simulink model "test_descramble_x_eng_reord"  (Simulink 6.2)
settings: Solver=ode45  StartTime=0.0  StopTime=10000  RelTol=1e-3
undefined symbols (not defined in the file or in its folder): BitWidth, cmult_4bit_em
libraries: xbsIndex_r3 x370, casper_library x29, xps_library x9, simulink x1
(part 2 of 3)

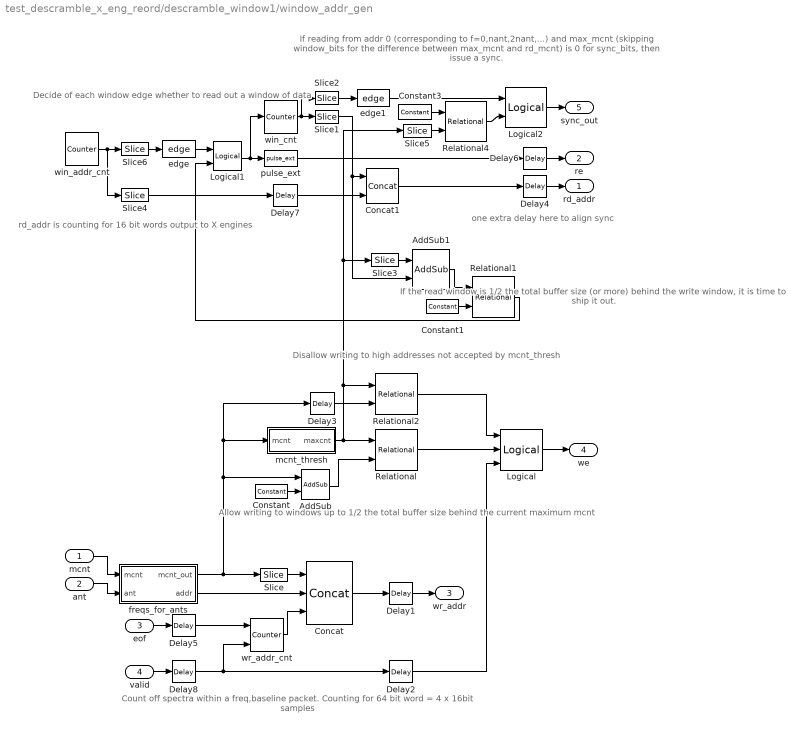
== system test_descramble_x_eng_reord/descramble_window1/window_addr_gen ==
  note: one extra delay
      | here to align sync
  note: If reading from addr 0 (corresponding to f=0,nant,2nant,...)
      | and max_mcnt (skipping window_bits for the difference
      | between max_mcnt and rd_mcnt) is 0 for sync_bits, then
      | issue a sync.
  note: Allow writing to windows
      | up to 1/2 the total buffer size
      |  behind the current maximum mcnt
  note: Count off spectra
      | within a freq,baseline
      | packet.  Counting for
      | 64 bit word = 4 x 16bit samples
  note: Decide of each window
      | edge whether to read
      | out a window of data
  note: If the read window is 1/2
      | the total buffer size (or more)
      | behind the write window,
      | it is time to ship it out.
  note: rd_addr is counting for
      | 16 bit words output to
      | X engines
  note: Disallow writing to high addresses
      | not accepted by mcnt_thresh
  mcnt : Inport  Port=1  LatchInput=off
  ant : Inport  Port=2  LatchInput=off
  eof : Inport  Port=3  LatchInput=off
  valid : Inport  Port=4  LatchInput=off
  AddSub : xbsIndex_r3/AddSub  mode=Addition  precision=User Defined  arith_type=Unsigned  n_bits=48 - ant_bits  bin_pt=0  quantization=Truncate  overflow=Wrap  latency=2  explicit_period=off  period=1  use_carryin=off  use_carryout=off  en=off  dbl_ovrd=off  show_param=off  use_core=on  pipeline=off  use_rpm=on  gen_core=off
      settings: xl_area=[0, 0, 0, 0, 0, 0, 0]
  AddSub1 : xbsIndex_r3/AddSub  mode=Subtraction  precision=User Defined  arith_type=Unsigned  n_bits=window_bits  bin_pt=0  quantization=Truncate  overflow=Wrap  latency=2  explicit_period=off  period=1  use_carryin=off  use_carryout=off  en=off  dbl_ovrd=off  show_param=off  use_core=on  pipeline=off  use_rpm=on  gen_core=off
      settings: xl_area=[0, 0, 0, 0, 0, 0, 0]
  Concat : xbsIndex_r3/Concat  num_inputs=3  explicit_period=off  period=1  dbl_ovrd=off
  Concat1 : xbsIndex_r3/Concat  num_inputs=2  explicit_period=off  period=1  dbl_ovrd=off
  Constant : xbsIndex_r3/Constant  const=2^(window_bits - 1)  equ=P=C  arith_type=Unsigned  n_bits=48 - ant_bits  bin_pt=0  opselect=C  inp2=PCIN>>17  opr=+  inp1=P  carry=CIN  iostate=0  explicit_period=on  period=1  dbl_ovrd=off
  Constant1 : xbsIndex_r3/Constant  const=2^(window_bits - 1)  equ=P=C  arith_type=Unsigned  n_bits=window_bits  bin_pt=0  opselect=C  inp2=PCIN>>17  opr=+  inp1=P  carry=CIN  iostate=0  explicit_period=on  period=1  dbl_ovrd=off
  Constant3 : xbsIndex_r3/Constant  const=0  equ=P=C  arith_type=Unsigned  n_bits=sync_bits - x_int_bits - ant_bits - window_bits  bin_pt=0  opselect=C  inp2=PCIN>>17  opr=+  inp1=P  carry=CIN  iostate=0  explicit_period=on  period=1  dbl_ovrd=off
  Delay1 : xbsIndex_r3/Delay  latency=3  reg_retiming=off  explicit_period=off  period=1  en=off  accept_only_valid=off  init_zero=on  dbl_ovrd=off  show_param=off
      settings: xl_area=[0, 0, 0, 0, 0, 0, 0]
  Delay2 : xbsIndex_r3/Delay  latency=3  reg_retiming=off  explicit_period=off  period=1  en=off  accept_only_valid=off  init_zero=on  dbl_ovrd=off  show_param=off
      settings: xl_area=[0, 0, 0, 0, 0, 0, 0]
  Delay3 : xbsIndex_r3/Delay  latency=2  reg_retiming=off  explicit_period=off  period=1  en=off  accept_only_valid=off  init_zero=on  dbl_ovrd=off  show_param=off
      settings: xl_area=[0, 0, 0, 0, 0, 0, 0]
  Delay{4..8} (5 alike) : xbsIndex_r3/Delay  latency=1  reg_retiming=off  explicit_period=off  period=1  en=off  accept_only_valid=off  init_zero=on  dbl_ovrd=off  show_param=off
      settings: xl_area=[0, 0, 0, 0, 0, 0, 0]
  Logical : xbsIndex_r3/Logical  logical_function=AND  inputs=3  precision=Full  arith_type=Unsigned  n_bits=8  bin_pt=2  align_bp=on  latency=0  explicit_period=off  period=1  en=off  dbl_ovrd=off  show_param=off
      settings: xl_area=[0, 0, 0, 0, 0, 0, 0]
  Logical1 : xbsIndex_r3/Logical  logical_function=AND  inputs=2  precision=Full  arith_type=Unsigned  n_bits=8  bin_pt=2  align_bp=on  latency=0  explicit_period=off  period=1  en=off  dbl_ovrd=off  show_param=off
      settings: xl_area=[0, 0, 0, 0, 0, 0, 0]
  Logical2 : xbsIndex_r3/Logical  logical_function=AND  inputs=2  precision=Full  arith_type=Unsigned  n_bits=8  bin_pt=2  align_bp=on  latency=0  explicit_period=off  period=1  en=off  dbl_ovrd=off  show_param=off
      settings: xl_area=[0, 0, 0, 0, 0, 0, 0]
  Relational : xbsIndex_r3/Relational  mode=a<b  latency=1  explicit_period=off  period=1  en=off  dbl_ovrd=off  show_param=off
      settings: xl_area=[0, 0, 0, 0, 0, 0, 0]
  Relational1 : xbsIndex_r3/Relational  mode=a>=b  latency=1  explicit_period=on  period=1  en=off  dbl_ovrd=off  show_param=off
      settings: xl_area=[0, 0, 0, 0, 0, 0, 0]
  Relational2 : xbsIndex_r3/Relational  mode=a>=b  latency=1  explicit_period=off  period=1  en=off  dbl_ovrd=off  show_param=off
      settings: xl_area=[0, 0, 0, 0, 0, 0, 0]
  Relational4 : xbsIndex_r3/Relational  mode=a=b  latency=1  explicit_period=off  period=1  en=off  dbl_ovrd=off  show_param=off
      settings: xl_area=[0, 0, 0, 0, 0, 0, 0]
  Slice : xbsIndex_r3/Slice  mode=Lower Bit Location + Width  nbits=window_bits  bit1=0  base1=MSB of Input  bit0=0  base0=LSB of Input  boolean_output=off  explicit_period=off  period=1  dbl_ovrd=off
  Slice1 : xbsIndex_r3/Slice  mode=Lower Bit Location + Width  nbits=window_bits  bit1=0  base1=MSB of Input  bit0=0  base0=LSB of Input  boolean_output=off  explicit_period=off  period=1  dbl_ovrd=off
  Slice2 : xbsIndex_r3/Slice  mode=Upper Bit Location + Width  nbits=1  bit1=0  base1=MSB of Input  bit0=0  base0=LSB of Input  boolean_output=on  explicit_period=off  period=1  dbl_ovrd=off
  Slice3 : xbsIndex_r3/Slice  mode=Lower Bit Location + Width  nbits=window_bits  bit1=0  base1=MSB of Input  bit0=0  base0=LSB of Input  boolean_output=off  explicit_period=off  period=1  dbl_ovrd=off
  Slice4 : xbsIndex_r3/Slice  mode=Lower Bit Location + Width  nbits=x_int_bits + ant_bits  bit1=0  base1=MSB of Input  bit0=0  base0=LSB of Input  boolean_output=off  explicit_period=off  period=1  dbl_ovrd=off
  Slice5 : xbsIndex_r3/Slice  mode=Two Bit Locations  nbits=window_bits  bit1=sync_bits - x_int_bits - ant_bits - 1  base1=LSB of Input  bit0=window_bits  base0=LSB of Input  boolean_output=off  explicit_period=off  period=1  dbl_ovrd=off
  Slice6 : xbsIndex_r3/Slice  mode=Upper Bit Location + Width  nbits=1  bit1=0  base1=MSB of Input  bit0=0  base0=LSB of Input  boolean_output=on  explicit_period=off  period=1  dbl_ovrd=off
  edge : casper_library/Misc/edge
  edge1 : casper_library/Misc/edge
  freqs_for_ants : Subsystem
  mcnt_thresh : Subsystem
  pulse_ext : casper_library/Misc/pulse_ext  pulse_len=2^(x_int_bits + ant_bits)
  win_addr_cnt : xbsIndex_r3/Counter  cnt_type=Free Running  n_bits=x_int_bits + ant_bits + 1  bin_pt=0  arith_type=Unsigned  start_count=0  cnt_to=Inf  cnt_by_val=1  operation=Up  explicit_period=off  period=1  load_pin=off  rst=off  en=off  dbl_ovrd=off  show_param=off  use_rpm=on  gen_core=off
      settings: xl_area=[0, 0, 0, 0, 0, 0, 0]
  win_cnt : xbsIndex_r3/Counter  cnt_type=Free Running  n_bits=window_bits + 1  bin_pt=0  arith_type=Unsigned  start_count=0  cnt_to=Inf  cnt_by_val=1  operation=Up  explicit_period=off  period=1  load_pin=off  rst=off  en=on  dbl_ovrd=off  show_param=off  use_rpm=on  gen_core=off
      settings: xl_area=[0, 0, 0, 0, 0, 0, 0]
  wr_addr_cnt : xbsIndex_r3/Counter  cnt_type=Free Running  n_bits=x_int_bits - 2  bin_pt=0  arith_type=Unsigned  start_count=0  cnt_to=Inf  cnt_by_val=1  operation=Up  explicit_period=off  period=1  load_pin=off  rst=on  en=on  dbl_ovrd=off  show_param=off  use_rpm=on  gen_core=off
      settings: xl_area=[0, 0, 0, 0, 0, 0, 0]
  rd_addr : Outport
  re : Outport  Port=2
  wr_addr : Outport  Port=3
  we : Outport  Port=4
  sync_out : Outport  Port=5
  wires:
  pulse_ext/1 -> Delay6/1
  Concat1/1 -> Delay4/1
  Delay7/1 -> Concat1/2
  Slice2/1 -> edge1/1
  Slice1/1 -> Concat1/1, AddSub1/2
  Slice4/1 -> Delay7/1
  freqs_for_ants/1(mcnt_out) -> Delay3/1, mcnt_thresh/1(mcnt), AddSub/1, Slice/1
  edge/1 -> Logical1/1
  Slice6/1 -> edge/1
  win_addr_cnt/1 -> Slice4/1, Slice6/1
  Delay6/1 -> re/1
  Delay4/1 -> rd_addr/1
  Relational1/1 -> Logical1/2
  Logical2/1 -> sync_out/1
  Relational4/1 -> Logical2/2
  Slice5/1 -> Relational4/2
  Constant3/1 -> Relational4/1
  edge1/1 -> Logical2/1
  Delay3/1 -> Relational2/2
  Relational2/1 -> Logical/1
  mcnt_thresh/1(maxcnt) -> Relational2/1, Slice5/1, Slice3/1, Relational/1
  Constant/1 -> AddSub/2
  mcnt/1 -> freqs_for_ants/1(mcnt)
  AddSub/1 -> Relational/2
  Slice/1 -> Concat/1
  freqs_for_ants/2(addr) -> Concat/2
  Concat/1 -> Delay1/1
  Delay1/1 -> wr_addr/1
  ant/1 -> freqs_for_ants/2(ant)
  wr_addr_cnt/1 -> Concat/3
  valid/1 -> Delay8/1
  eof/1 -> Delay5/1
  Relational/1 -> Logical/2
  Logical/1 -> we/1
  Delay2/1 -> Logical/3
  Logical1/1 -> win_cnt/1, pulse_ext/1
  Slice3/1 -> AddSub1/1
  win_cnt/1 -> Slice2/1, Slice1/1
  AddSub1/1 -> Relational1/1
  Constant1/1 -> Relational1/2
  Delay5/1 -> wr_addr_cnt/1
  Delay8/1 -> wr_addr_cnt/2, Delay2/1

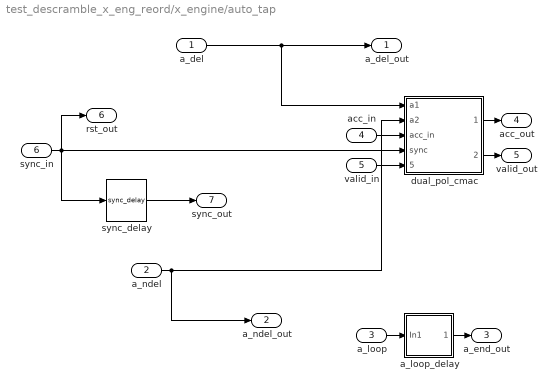
== system test_descramble_x_eng_reord/x_engine/auto_tap ==
  a_del : Inport  Port=1  LatchInput=off
  a_ndel : Inport  Port=2  LatchInput=off
  a_loop : Inport  Port=3  LatchInput=off
  acc_in : Inport  Port=4  LatchInput=off
  valid_in : Inport  Port=5  LatchInput=off
  sync_in : Inport  Port=6  LatchInput=off
  a_loop_delay : Subsystem  BlockChoice=delay_bram
      link override delay_bram: DelayLen=(acc_len - 1)*ceil(n_ants/2) + ceil(n_ants/2)-floor(n_ants/2)  bram_latency=bram_latency
      link override delay_bram/Constant2: equ=P=C
      settings: AttributesFormatString=%<BlockChoice>  TemplateBlock=casper_library/Delays/delay  MemberBlocks=delay_bram,delay_slr
  dual_pol_cmac : Subsystem
  sync_delay : casper_library/Delays/sync_delay  DelayLen=add_latency + mult_latency + acc_len + floor(n_ants/2 + 1) + 1
      link override Constant: equ=P=C
      link override Constant1: equ=P=C
      link override Constant2: equ=P=C
      link override Constant3: equ=P=C
  a_del_out : Outport
  a_ndel_out : Outport  Port=2
  a_end_out : Outport  Port=3
  acc_out : Outport  Port=4
  valid_out : Outport  Port=5
  rst_out : Outport  Port=6
  sync_out : Outport  Port=7
  wires:
  sync_in/1 -> sync_delay/1, dual_pol_cmac/4(sync), rst_out/1
  a_del/1 -> dual_pol_cmac/1(a1), a_del_out/1
  dual_pol_cmac/1(acc_out) -> acc_out/1
  acc_in/1 -> dual_pol_cmac/3(acc_in)
  dual_pol_cmac/2(valid_out) -> valid_out/1
  valid_in/1 -> dual_pol_cmac/5(valid_in)
  a_ndel/1 -> dual_pol_cmac/2(a2), a_ndel_out/1
  a_loop/1 -> a_loop_delay/1(In1)
  a_loop_delay/1(Out1) -> a_end_out/1
  sync_delay/1 -> sync_out/1

== system test_descramble_x_eng_reord/descramble_window1/window_addr_gen/freqs_for_ants ==
  note: skip bits of mcnt
      | for frequencies sent
      | to other X engines
  note: If correlator is configured to do fewer antennas, then more
      | frequencies come.  We just pretend here that the extra
      | frequencies are other antennas.
  mcnt : Inport  Port=1  LatchInput=off
  ant : Inport  Port=2  LatchInput=off
  Concat3 : xbsIndex_r3/Concat  num_inputs=2  explicit_period=off  period=1  dbl_ovrd=off
  Slice1 : xbsIndex_r3/Slice  mode=Lower Bit Location + Width  nbits=ant_bits  bit1=0  base1=MSB of Input  bit0=0  base0=LSB of Input  boolean_output=off  explicit_period=off  period=1  dbl_ovrd=off
  Slice14 : xbsIndex_r3/Slice  mode=Two Bit Locations  nbits=ant_bits  bit1=0  base1=MSB of Input  bit0=ant_bits  base0=LSB of Input  boolean_output=off  explicit_period=off  period=1  dbl_ovrd=off
  Slice18 : xbsIndex_r3/Slice  mode=Lower Bit Location + Width  nbits=ant_bits  bit1=0  base1=MSB of Input  bit0=0  base0=LSB of Input  boolean_output=off  explicit_period=off  period=1  dbl_ovrd=off
  Slice19 : xbsIndex_r3/Slice  mode=Two Bit Locations  nbits=48  bit1=0  base1=MSB of Input  bit0=ant_bits  base0=LSB of Input  boolean_output=off  explicit_period=off  period=1  dbl_ovrd=off
  mcnt_out : Outport
  addr : Outport  Port=2
  wires:
  Slice19/1 -> mcnt_out/1
  Slice18/1 -> addr/1
  Slice14/1 -> Concat3/1
  Slice1/1 -> Concat3/2
  Concat3/1 -> Slice19/1, Slice18/1
  ant/1 -> Slice1/1
  mcnt/1 -> Slice14/1

== system test_descramble_x_eng_reord/descramble_window1/window_addr_gen/mcnt_thresh ==
  note: timeout of a bad
      | master count
      | in ~2^20 clocks
  note: capture any new mcnts
      | which are within 1/4 buffer
      | of the previous mcnt.
      | This prevents locking onto
      | bad mcnts
  mcnt : Inport  Port=1  LatchInput=off
  AddSub : xbsIndex_r3/AddSub  mode=Addition  precision=User Defined  arith_type=Unsigned  n_bits=48 - ant_bits  bin_pt=0  quantization=Truncate  overflow=Wrap  latency=2  explicit_period=off  period=1  use_carryin=off  use_carryout=off  en=off  dbl_ovrd=off  show_param=off  use_core=on  pipeline=off  use_rpm=on  gen_core=off
      settings: xl_area=[0, 0, 0, 0, 0, 0, 0]
  Constant : xbsIndex_r3/Constant  const=2^(window_bits - 2)  equ=P=C  arith_type=Unsigned  n_bits=48 - ant_bits  bin_pt=0  opselect=C  inp2=PCIN>>17  opr=+  inp1=P  carry=CIN  iostate=0  explicit_period=on  period=1  dbl_ovrd=off
  Counter : xbsIndex_r3/Counter  cnt_type=Free Running  n_bits=21  bin_pt=0  arith_type=Unsigned  start_count=0  cnt_to=Inf  cnt_by_val=1  operation=Up  explicit_period=on  period=1  load_pin=off  rst=on  en=off  dbl_ovrd=off  show_param=off  use_rpm=on  gen_core=off
      settings: xl_area=[0, 0, 0, 0, 0, 0, 0]
  Delay : xbsIndex_r3/Delay  latency=2  reg_retiming=off  explicit_period=off  period=1  en=off  accept_only_valid=off  init_zero=on  dbl_ovrd=off  show_param=off
      settings: xl_area=[0, 0, 0, 0, 0, 0, 0]
  Delay1 : xbsIndex_r3/Delay  latency=1  reg_retiming=off  explicit_period=off  period=1  en=off  accept_only_valid=off  init_zero=on  dbl_ovrd=off  show_param=off
      settings: xl_area=[0, 0, 0, 0, 0, 0, 0]
  Logical : xbsIndex_r3/Logical  logical_function=AND  inputs=2  precision=Full  arith_type=Unsigned  n_bits=8  bin_pt=2  align_bp=on  latency=0  explicit_period=off  period=1  en=off  dbl_ovrd=off  show_param=off
      settings: xl_area=[0, 0, 0, 0, 0, 0, 0]
  Logical1 : xbsIndex_r3/Logical  logical_function=OR  inputs=2  precision=Full  arith_type=Unsigned  n_bits=8  bin_pt=2  align_bp=on  latency=0  explicit_period=off  period=1  en=off  dbl_ovrd=off  show_param=off
      settings: xl_area=[0, 0, 0, 0, 0, 0, 0]
  Register : xbsIndex_r3/Register  init=0  reg_only_valid=off  explicit_period=on  period=1  rst=off  en=on  out_en=off  dbl_ovrd=off  show_param=off
      settings: xl_area=[0, 0, 0, 0, 0, 0, 0]
  Relational : xbsIndex_r3/Relational  mode=a>b  latency=1  explicit_period=off  period=1  en=off  dbl_ovrd=off  show_param=off
      settings: xl_area=[0, 0, 0, 0, 0, 0, 0]
  Relational1 : xbsIndex_r3/Relational  mode=a<b  latency=1  explicit_period=off  period=1  en=off  dbl_ovrd=off  show_param=off
      settings: xl_area=[0, 0, 0, 0, 0, 0, 0]
  Slice : xbsIndex_r3/Slice  mode=Upper Bit Location + Width  nbits=1  bit1=0  base1=MSB of Input  bit0=0  base0=LSB of Input  boolean_output=on  explicit_period=off  period=1  dbl_ovrd=off
  maxcnt : Outport
  wires:
  Constant/1 -> AddSub/2
  Register/1 -> AddSub/1, Delay/1, maxcnt/1
  AddSub/1 -> Relational1/2
  Relational/1 -> Logical/1
  Counter/1 -> Slice/1
  Logical/1 -> Logical1/2
  Logical1/1 -> Counter/1, Register/2
  Slice/1 -> Logical1/1
  Delay/1 -> Relational/2
  mcnt/1 -> Relational/1, Relational1/1, Delay1/1
  Relational1/1 -> Logical/2
  Delay1/1 -> Register/1

== system test_descramble_x_eng_reord/x_engine/auto_tap/a_loop_delay ==
  In1 : Inport  Port=1  LatchInput=off
  delay_bram : casper_library/Delays/delay_bram  DelayLen=(acc_len - 1)*ceil(n_ants/2) + ceil(n_ants/2)-floor(n_ants/2)  bram_latency=bram_latency
  Out1 : Outport
  wires:
  In1/1 -> delay_bram/1
  delay_bram/1 -> Out1/1

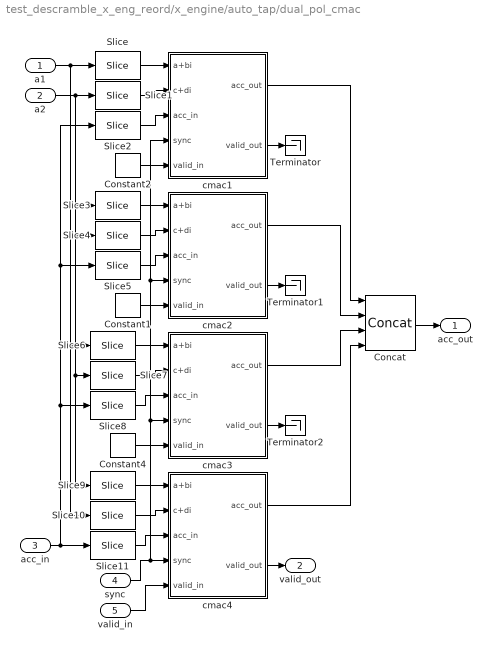
== system test_descramble_x_eng_reord/x_engine/auto_tap/dual_pol_cmac ==
  a1 : Inport  Port=1  LatchInput=off
  a2 : Inport  Port=2  LatchInput=off
  acc_in : Inport  Port=3  LatchInput=off
  sync : Inport  Port=4  LatchInput=off
  valid_in : Inport  Port=5  LatchInput=off
  Concat : xbsIndex_r3/Concat  num_inputs=4  explicit_period=off  period=1  dbl_ovrd=off
  Constant1 : xbsIndex_r3/Constant  const=0  equ=P=C  arith_type=Unsigned  n_bits=1  bin_pt=0  opselect=C  inp2=PCIN>>17  opr=+  inp1=P  carry=CIN  iostate=0  explicit_period=off  period=1  dbl_ovrd=off
  Constant2 : xbsIndex_r3/Constant  const=0  equ=P=C  arith_type=Unsigned  n_bits=1  bin_pt=0  opselect=C  inp2=PCIN>>17  opr=+  inp1=P  carry=CIN  iostate=0  explicit_period=off  period=1  dbl_ovrd=off
  Constant4 : xbsIndex_r3/Constant  const=0  equ=P=C  arith_type=Unsigned  n_bits=1  bin_pt=0  opselect=C  inp2=PCIN>>17  opr=+  inp1=P  carry=CIN  iostate=0  explicit_period=off  period=1  dbl_ovrd=off
  Slice{,1,6,9} (4 alike) : xbsIndex_r3/Slice  mode=Upper Bit Location + Width  nbits=2*n_bits  bit1=0  base1=MSB of Input  bit0=0  base0=LSB of Input  boolean_output=off  explicit_period=off  period=1  dbl_ovrd=off
  Slice{3..4,7,10} (4 alike) : xbsIndex_r3/Slice  mode=Upper Bit Location + Width  nbits=2*n_bits  bit1=-2*n_bits  base1=MSB of Input  bit0=0  base0=LSB of Input  boolean_output=off  explicit_period=off  period=1  dbl_ovrd=off
  Slice11 : xbsIndex_r3/Slice  mode=Upper Bit Location + Width  nbits=2*n_bits_out  bit1=-6*n_bits_out  base1=MSB of Input  bit0=0  base0=LSB of Input  boolean_output=off  explicit_period=off  period=1  dbl_ovrd=off
  Slice2 : xbsIndex_r3/Slice  mode=Upper Bit Location + Width  nbits=2*n_bits_out  bit1=0  base1=MSB of Input  bit0=0  base0=LSB of Input  boolean_output=off  explicit_period=off  period=1  dbl_ovrd=off
  Slice5 : xbsIndex_r3/Slice  mode=Upper Bit Location + Width  nbits=2*n_bits_out  bit1=-2*n_bits_out  base1=MSB of Input  bit0=0  base0=LSB of Input  boolean_output=off  explicit_period=off  period=1  dbl_ovrd=off
  Slice8 : xbsIndex_r3/Slice  mode=Upper Bit Location + Width  nbits=2*n_bits_out  bit1=-4*n_bits_out  base1=MSB of Input  bit0=0  base0=LSB of Input  boolean_output=off  explicit_period=off  period=1  dbl_ovrd=off
  Terminator : Terminator
  Terminator1 : Terminator
  Terminator2 : Terminator
  cmac1 : Subsystem
  cmac2 : Subsystem
  cmac3 : Subsystem
  cmac4 : Subsystem
  acc_out : Outport
  valid_out : Outport  Port=2
  wires:
  acc_in/1 -> Slice2/1, Slice5/1, Slice8/1, Slice11/1
  a2/1 -> Slice9/1, Slice7/1, Slice4/1, Slice1/1
  a1/1 -> Slice10/1, Slice6/1, Slice3/1, Slice/1
  cmac4/1(acc_out) -> Concat/4
  cmac3/1(acc_out) -> Concat/3
  cmac2/1(acc_out) -> Concat/2
  cmac1/1(acc_out) -> Concat/1
  cmac4/2(valid_out) -> valid_out/1
  cmac3/2(valid_out) -> Terminator2/1
  cmac2/2(valid_out) -> Terminator1/1
  sync/1 -> cmac1/4(sync), cmac2/4(sync), cmac3/4(sync), cmac4/4(sync)
  valid_in/1 -> cmac4/5(valid_in)
  Slice11/1 -> cmac4/3(acc_in)
  Slice10/1 -> cmac4/2(c+di)
  Slice9/1 -> cmac4/1(a+bi)
  Constant4/1 -> cmac3/5(valid_in)
  Slice8/1 -> cmac3/3(acc_in)
  Slice7/1 -> cmac3/2(c+di)
  Slice6/1 -> cmac3/1(a+bi)
  Constant1/1 -> cmac2/5(valid_in)
  cmac1/2(valid_out) -> Terminator/1
  Constant2/1 -> cmac1/5(valid_in)
  Concat/1 -> acc_out/1
  Slice5/1 -> cmac2/3(acc_in)
  Slice4/1 -> cmac2/2(c+di)
  Slice3/1 -> cmac2/1(a+bi)
  Slice2/1 -> cmac1/3(acc_in)
  Slice1/1 -> cmac1/2(c+di)
  Slice/1 -> cmac1/1(a+bi)

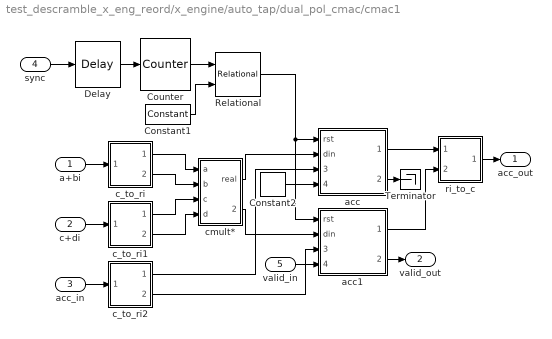
== system test_descramble_x_eng_reord/x_engine/auto_tap/dual_pol_cmac/cmac1 ==
  a+bi : Inport  Port=1  LatchInput=off
  c+di : Inport  Port=2  LatchInput=off
  acc_in : Inport  Port=3  LatchInput=off
  sync : Inport  Port=4  LatchInput=off
  valid_in : Inport  Port=5  LatchInput=off
  Constant1 : xbsIndex_r3/Constant  const=0  equ=P=C  arith_type=Unsigned  n_bits=bit_growth  bin_pt=0  opselect=C  inp2=PCIN>>17  opr=+  inp1=P  carry=CIN  iostate=0  explicit_period=off  period=1  dbl_ovrd=off
  Constant2 : xbsIndex_r3/Constant  const=0  equ=P=C  arith_type=Unsigned  n_bits=1  bin_pt=0  opselect=C  inp2=PCIN>>17  opr=+  inp1=P  carry=CIN  iostate=0  explicit_period=off  period=1  dbl_ovrd=off
  Counter : xbsIndex_r3/Counter  cnt_type=Count Limited  n_bits=bit_growth  bin_pt=0  arith_type=Unsigned  start_count=0  cnt_to=acc_len - 1  cnt_by_val=1  operation=Up  explicit_period=off  period=1  load_pin=off  rst=on  en=off  dbl_ovrd=off  show_param=off  use_rpm=on  gen_core=off
      settings: xl_area=[0, 0, 0, 0, 0, 0, 0]
  Delay : xbsIndex_r3/Delay  latency=add_latency + mult_latency - 1  reg_retiming=off  explicit_period=off  period=1  en=off  accept_only_valid=off  init_zero=on  dbl_ovrd=off  show_param=off
      settings: xl_area=[0, 0, 0, 0, 0, 0, 0]
  Relational : xbsIndex_r3/Relational  mode=a=b  latency=1  explicit_period=off  period=1  en=off  dbl_ovrd=off  show_param=off
      settings: xl_area=[0, 0, 0, 0, 0, 0, 0]
  Terminator : Terminator
  acc : Subsystem
  acc1 : Subsystem
  c_to_ri : Subsystem
  c_to_ri1 : Subsystem
  c_to_ri2 : Subsystem
  cmult* : Subsystem  BlockChoice=cmult_4bit_em*
      link override cmult_4bit_br*: mult_latency=mult_latency  add_latency=add_latency
      link override cmult_4bit_em*: mult_latency=mult_latency  add_latency=add_latency
      link override cmult_4bit_sl*: mult_latency=mult_latency  add_latency=add_latency
      settings: AttributesFormatString=%<BlockChoice>  TemplateBlock=casper_library/Multipliers/cmult*  MemberBlocks=cmult_4bit_br*,cmult_4bit_em*,cmult_4bit_sl*
      mask Type: cmult*
  ri_to_c : Subsystem
  acc_out : Outport
  valid_out : Outport  Port=2
  wires:
  valid_in/1 -> acc1/4(valid_in)
  acc1/2(valid_out) -> valid_out/1
  acc/2(valid_out) -> Terminator/1
  Constant2/1 -> acc/4(valid_in)
  Delay/1 -> Counter/1
  sync/1 -> Delay/1
  Constant1/1 -> Relational/2
  Counter/1 -> Relational/1
  Relational/1 -> acc1/1(rst), acc/1(rst)
  c_to_ri2/2(Out2) -> acc1/3(acc_in)
  c_to_ri2/1(Out1) -> acc/3(acc_in)
  ri_to_c/1(Out1) -> acc_out/1
  acc1/1(acc_out) -> ri_to_c/2(In2)
  acc/1(acc_out) -> ri_to_c/1(In1)
  acc_in/1 -> c_to_ri2/1(In1)
  c_to_ri1/2(Out2) -> cmult*/4(d)
  c_to_ri1/1(Out1) -> cmult*/3(c)
  c+di/1 -> c_to_ri1/1(In1)
  c_to_ri/2(Out2) -> cmult*/2(b)
  c_to_ri/1(Out1) -> cmult*/1(a)
  a+bi/1 -> c_to_ri/1(In1)
  cmult*/2(imag) -> acc1/2(din)
  cmult*/1(real) -> acc/2(din)

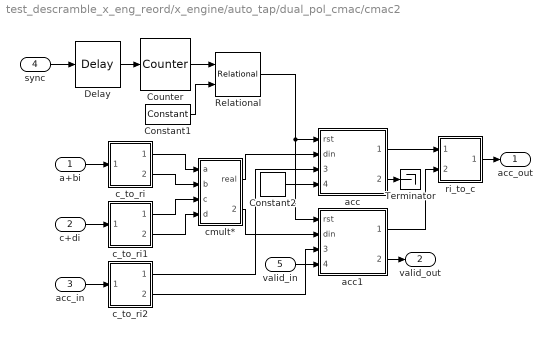
== system test_descramble_x_eng_reord/x_engine/auto_tap/dual_pol_cmac/cmac2 ==
  a+bi : Inport  Port=1  LatchInput=off
  c+di : Inport  Port=2  LatchInput=off
  acc_in : Inport  Port=3  LatchInput=off
  sync : Inport  Port=4  LatchInput=off
  valid_in : Inport  Port=5  LatchInput=off
  Constant1 : xbsIndex_r3/Constant  const=0  equ=P=C  arith_type=Unsigned  n_bits=bit_growth  bin_pt=0  opselect=C  inp2=PCIN>>17  opr=+  inp1=P  carry=CIN  iostate=0  explicit_period=off  period=1  dbl_ovrd=off
  Constant2 : xbsIndex_r3/Constant  const=0  equ=P=C  arith_type=Unsigned  n_bits=1  bin_pt=0  opselect=C  inp2=PCIN>>17  opr=+  inp1=P  carry=CIN  iostate=0  explicit_period=off  period=1  dbl_ovrd=off
  Counter : xbsIndex_r3/Counter  cnt_type=Count Limited  n_bits=bit_growth  bin_pt=0  arith_type=Unsigned  start_count=0  cnt_to=acc_len - 1  cnt_by_val=1  operation=Up  explicit_period=off  period=1  load_pin=off  rst=on  en=off  dbl_ovrd=off  show_param=off  use_rpm=on  gen_core=off
      settings: xl_area=[0, 0, 0, 0, 0, 0, 0]
  Delay : xbsIndex_r3/Delay  latency=add_latency + mult_latency - 1  reg_retiming=off  explicit_period=off  period=1  en=off  accept_only_valid=off  init_zero=on  dbl_ovrd=off  show_param=off
      settings: xl_area=[0, 0, 0, 0, 0, 0, 0]
  Relational : xbsIndex_r3/Relational  mode=a=b  latency=1  explicit_period=off  period=1  en=off  dbl_ovrd=off  show_param=off
      settings: xl_area=[0, 0, 0, 0, 0, 0, 0]
  Terminator : Terminator
  acc : Subsystem
  acc1 : Subsystem
  c_to_ri : Subsystem
  c_to_ri1 : Subsystem
  c_to_ri2 : Subsystem
  cmult* : Subsystem  BlockChoice=cmult_4bit_em*
      link override cmult_4bit_br*: mult_latency=mult_latency  add_latency=add_latency
      link override cmult_4bit_em*: mult_latency=mult_latency  add_latency=add_latency
      link override cmult_4bit_sl*: mult_latency=mult_latency  add_latency=add_latency
      settings: AttributesFormatString=%<BlockChoice>  TemplateBlock=casper_library/Multipliers/cmult*  MemberBlocks=cmult_4bit_br*,cmult_4bit_em*,cmult_4bit_sl*
      mask Type: cmult*
  ri_to_c : Subsystem
  acc_out : Outport
  valid_out : Outport  Port=2
  wires:
  cmult*/1(real) -> acc/2(din)
  cmult*/2(imag) -> acc1/2(din)
  a+bi/1 -> c_to_ri/1(In1)
  c_to_ri/1(Out1) -> cmult*/1(a)
  c_to_ri/2(Out2) -> cmult*/2(b)
  c+di/1 -> c_to_ri1/1(In1)
  c_to_ri1/1(Out1) -> cmult*/3(c)
  c_to_ri1/2(Out2) -> cmult*/4(d)
  acc_in/1 -> c_to_ri2/1(In1)
  acc/1(acc_out) -> ri_to_c/1(In1)
  acc1/1(acc_out) -> ri_to_c/2(In2)
  ri_to_c/1(Out1) -> acc_out/1
  c_to_ri2/1(Out1) -> acc/3(acc_in)
  c_to_ri2/2(Out2) -> acc1/3(acc_in)
  Relational/1 -> acc/1(rst), acc1/1(rst)
  Counter/1 -> Relational/1
  Constant1/1 -> Relational/2
  sync/1 -> Delay/1
  Delay/1 -> Counter/1
  Constant2/1 -> acc/4(valid_in)
  acc/2(valid_out) -> Terminator/1
  acc1/2(valid_out) -> valid_out/1
  valid_in/1 -> acc1/4(valid_in)

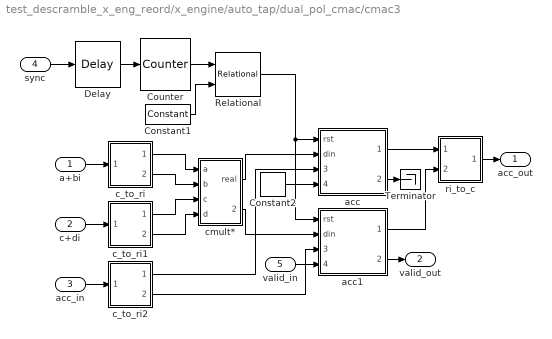
== system test_descramble_x_eng_reord/x_engine/auto_tap/dual_pol_cmac/cmac3 ==
  a+bi : Inport  Port=1  LatchInput=off
  c+di : Inport  Port=2  LatchInput=off
  acc_in : Inport  Port=3  LatchInput=off
  sync : Inport  Port=4  LatchInput=off
  valid_in : Inport  Port=5  LatchInput=off
  Constant1 : xbsIndex_r3/Constant  const=0  equ=P=C  arith_type=Unsigned  n_bits=bit_growth  bin_pt=0  opselect=C  inp2=PCIN>>17  opr=+  inp1=P  carry=CIN  iostate=0  explicit_period=off  period=1  dbl_ovrd=off
  Constant2 : xbsIndex_r3/Constant  const=0  equ=P=C  arith_type=Unsigned  n_bits=1  bin_pt=0  opselect=C  inp2=PCIN>>17  opr=+  inp1=P  carry=CIN  iostate=0  explicit_period=off  period=1  dbl_ovrd=off
  Counter : xbsIndex_r3/Counter  cnt_type=Count Limited  n_bits=bit_growth  bin_pt=0  arith_type=Unsigned  start_count=0  cnt_to=acc_len - 1  cnt_by_val=1  operation=Up  explicit_period=off  period=1  load_pin=off  rst=on  en=off  dbl_ovrd=off  show_param=off  use_rpm=on  gen_core=off
      settings: xl_area=[0, 0, 0, 0, 0, 0, 0]
  Delay : xbsIndex_r3/Delay  latency=add_latency + mult_latency - 1  reg_retiming=off  explicit_period=off  period=1  en=off  accept_only_valid=off  init_zero=on  dbl_ovrd=off  show_param=off
      settings: xl_area=[0, 0, 0, 0, 0, 0, 0]
  Relational : xbsIndex_r3/Relational  mode=a=b  latency=1  explicit_period=off  period=1  en=off  dbl_ovrd=off  show_param=off
      settings: xl_area=[0, 0, 0, 0, 0, 0, 0]
  Terminator : Terminator
  acc : Subsystem
  acc1 : Subsystem
  c_to_ri : Subsystem
  c_to_ri1 : Subsystem
  c_to_ri2 : Subsystem
  cmult* : Subsystem  BlockChoice=cmult_4bit_em*
      link override cmult_4bit_br*: mult_latency=mult_latency  add_latency=add_latency
      link override cmult_4bit_em*: mult_latency=mult_latency  add_latency=add_latency
      link override cmult_4bit_sl*: mult_latency=mult_latency  add_latency=add_latency
      settings: AttributesFormatString=%<BlockChoice>  TemplateBlock=casper_library/Multipliers/cmult*  MemberBlocks=cmult_4bit_br*,cmult_4bit_em*,cmult_4bit_sl*
      mask Type: cmult*
  ri_to_c : Subsystem
  acc_out : Outport
  valid_out : Outport  Port=2
  wires:
  cmult*/1(real) -> acc/2(din)
  cmult*/2(imag) -> acc1/2(din)
  a+bi/1 -> c_to_ri/1(In1)
  c_to_ri/1(Out1) -> cmult*/1(a)
  c_to_ri/2(Out2) -> cmult*/2(b)
  c+di/1 -> c_to_ri1/1(In1)
  c_to_ri1/1(Out1) -> cmult*/3(c)
  c_to_ri1/2(Out2) -> cmult*/4(d)
  acc_in/1 -> c_to_ri2/1(In1)
  acc/1(acc_out) -> ri_to_c/1(In1)
  acc1/1(acc_out) -> ri_to_c/2(In2)
  ri_to_c/1(Out1) -> acc_out/1
  c_to_ri2/1(Out1) -> acc/3(acc_in)
  c_to_ri2/2(Out2) -> acc1/3(acc_in)
  Relational/1 -> acc/1(rst), acc1/1(rst)
  Counter/1 -> Relational/1
  Constant1/1 -> Relational/2
  sync/1 -> Delay/1
  Delay/1 -> Counter/1
  Constant2/1 -> acc/4(valid_in)
  acc/2(valid_out) -> Terminator/1
  acc1/2(valid_out) -> valid_out/1
  valid_in/1 -> acc1/4(valid_in)

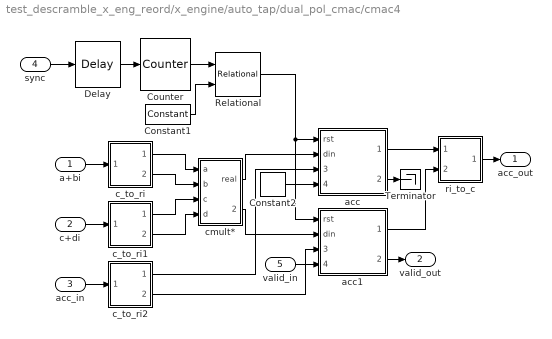
== system test_descramble_x_eng_reord/x_engine/auto_tap/dual_pol_cmac/cmac4 ==
  a+bi : Inport  Port=1  LatchInput=off
  c+di : Inport  Port=2  LatchInput=off
  acc_in : Inport  Port=3  LatchInput=off
  sync : Inport  Port=4  LatchInput=off
  valid_in : Inport  Port=5  LatchInput=off
  Constant1 : xbsIndex_r3/Constant  const=0  equ=P=C  arith_type=Unsigned  n_bits=bit_growth  bin_pt=0  opselect=C  inp2=PCIN>>17  opr=+  inp1=P  carry=CIN  iostate=0  explicit_period=off  period=1  dbl_ovrd=off
  Constant2 : xbsIndex_r3/Constant  const=0  equ=P=C  arith_type=Unsigned  n_bits=1  bin_pt=0  opselect=C  inp2=PCIN>>17  opr=+  inp1=P  carry=CIN  iostate=0  explicit_period=off  period=1  dbl_ovrd=off
  Counter : xbsIndex_r3/Counter  cnt_type=Count Limited  n_bits=bit_growth  bin_pt=0  arith_type=Unsigned  start_count=0  cnt_to=acc_len - 1  cnt_by_val=1  operation=Up  explicit_period=off  period=1  load_pin=off  rst=on  en=off  dbl_ovrd=off  show_param=off  use_rpm=on  gen_core=off
      settings: xl_area=[0, 0, 0, 0, 0, 0, 0]
  Delay : xbsIndex_r3/Delay  latency=add_latency + mult_latency - 1  reg_retiming=off  explicit_period=off  period=1  en=off  accept_only_valid=off  init_zero=on  dbl_ovrd=off  show_param=off
      settings: xl_area=[0, 0, 0, 0, 0, 0, 0]
  Relational : xbsIndex_r3/Relational  mode=a=b  latency=1  explicit_period=off  period=1  en=off  dbl_ovrd=off  show_param=off
      settings: xl_area=[0, 0, 0, 0, 0, 0, 0]
  Terminator : Terminator
  acc : Subsystem
  acc1 : Subsystem
  c_to_ri : Subsystem
  c_to_ri1 : Subsystem
  c_to_ri2 : Subsystem
  cmult* : Subsystem  BlockChoice=cmult_4bit_em*
      link override cmult_4bit_br*: mult_latency=mult_latency  add_latency=add_latency
      link override cmult_4bit_em*: mult_latency=mult_latency  add_latency=add_latency
      link override cmult_4bit_sl*: mult_latency=mult_latency  add_latency=add_latency
      settings: AttributesFormatString=%<BlockChoice>  TemplateBlock=casper_library/Multipliers/cmult*  MemberBlocks=cmult_4bit_br*,cmult_4bit_em*,cmult_4bit_sl*
      mask Type: cmult*
  ri_to_c : Subsystem
  acc_out : Outport
  valid_out : Outport  Port=2
  wires:
  cmult*/1(real) -> acc/2(din)
  cmult*/2(imag) -> acc1/2(din)
  a+bi/1 -> c_to_ri/1(In1)
  c_to_ri/1(Out1) -> cmult*/1(a)
  c_to_ri/2(Out2) -> cmult*/2(b)
  c+di/1 -> c_to_ri1/1(In1)
  c_to_ri1/1(Out1) -> cmult*/3(c)
  c_to_ri1/2(Out2) -> cmult*/4(d)
  acc_in/1 -> c_to_ri2/1(In1)
  acc/1(acc_out) -> ri_to_c/1(In1)
  acc1/1(acc_out) -> ri_to_c/2(In2)
  ri_to_c/1(Out1) -> acc_out/1
  c_to_ri2/1(Out1) -> acc/3(acc_in)
  c_to_ri2/2(Out2) -> acc1/3(acc_in)
  Relational/1 -> acc/1(rst), acc1/1(rst)
  Counter/1 -> Relational/1
  Constant1/1 -> Relational/2
  sync/1 -> Delay/1
  Delay/1 -> Counter/1
  Constant2/1 -> acc/4(valid_in)
  acc/2(valid_out) -> Terminator/1
  acc1/2(valid_out) -> valid_out/1
  valid_in/1 -> acc1/4(valid_in)

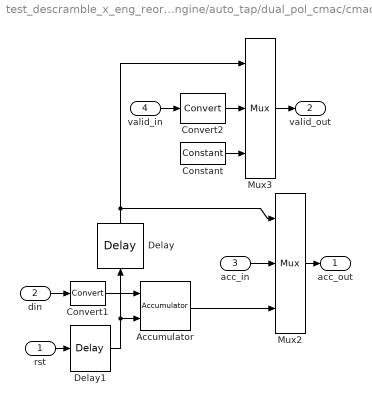
== system test_descramble_x_eng_reord/x_engine/auto_tap/dual_pol_cmac/cmac1/acc ==
  rst : Inport  Port=1  LatchInput=off
  din : Inport  Port=2  LatchInput=off
  acc_in : Inport  Port=3  LatchInput=off
  valid_in : Inport  Port=4  LatchInput=off
  Accumulator : xbsIndex_r3/Accumulator  n_bits=n_bits_out  overflow=Wrap  operation=Add  scale=1  explicit_period=on  period=1  rst=on  hasbypass=on  en=off  dbl_ovrd=off  show_param=off  gen_core=off  use_rpm=on
      settings: xl_area=[0, 0, 0, 0, 0, 0, 0]
  Constant : xbsIndex_r3/Constant  const=1  equ=P=C  arith_type=Boolean  n_bits=1  bin_pt=0  opselect=C  inp2=PCIN>>17  opr=+  inp1=P  carry=CIN  iostate=0  explicit_period=on  period=1  dbl_ovrd=off
  Convert1 : xbsIndex_r3/Convert  arith_type="Signed  (2's comp)"  n_bits=n_bits_out  bin_pt=2*(n_bits-1)  quantization=Truncate  overflow=Wrap  latency=0  explicit_period=off  period=1  dbl_ovrd=off  show_param=on  inserted_by_tool=off  pipeline=off
      settings: xl_area=[0, 0, 0, 0, 0, 0, 0]
  Convert2 : xbsIndex_r3/Convert  arith_type=Boolean  n_bits=8  bin_pt=6  quantization=Truncate  overflow=Wrap  latency=0  explicit_period=off  period=1  dbl_ovrd=off  show_param=off  inserted_by_tool=off  pipeline=off
      settings: xl_area=[0, 0, 0, 0, 0, 0, 0]
  Delay : xbsIndex_r3/Delay  Orientation=up  latency=0  reg_retiming=off  explicit_period=off  period=1  en=off  accept_only_valid=off  init_zero=on  dbl_ovrd=off  show_param=off
      settings: xl_area=[0, 0, 0, 0, 0, 0, 0]
  Delay1 : xbsIndex_r3/Delay  latency=0  reg_retiming=off  explicit_period=off  period=1  en=off  accept_only_valid=off  init_zero=on  dbl_ovrd=off  show_param=off
      settings: xl_area=[0, 0, 0, 0, 0, 0, 0]
  Mux2 : xbsIndex_r3/Mux  inputs=2  precision=Full  arith_type="Signed  (2's comp)"  n_bits=0  bin_pt=0  quantization="Round  (unbiased: +/- Inf)"  overflow=Wrap  latency=2  explicit_period=on  period=1  en=off  dbl_ovrd=off  show_param=off  mux_type=off  use_rpm=off  gen_core=off
      settings: xl_area=[0, 0, 0, 0, 0, 0, 0]
  Mux3 : xbsIndex_r3/Mux  inputs=2  precision=Full  arith_type="Signed  (2's comp)"  n_bits=0  bin_pt=0  quantization=Truncate  overflow=Wrap  latency=2  explicit_period=on  period=1  en=off  dbl_ovrd=off  show_param=off  mux_type=off  use_rpm=off  gen_core=off
      settings: xl_area=[0, 0, 0, 0, 0, 0, 0]
  acc_out : Outport
  valid_out : Outport  Port=2
  wires:
  Accumulator/1 -> Mux2/3
  Mux2/1 -> acc_out/1
  acc_in/1 -> Mux2/2
  valid_in/1 -> Convert2/1
  Constant/1 -> Mux3/3
  Mux3/1 -> valid_out/1
  din/1 -> Convert1/1
  rst/1 -> Delay1/1
  Delay/1 -> Mux3/1, Mux2/1
  Convert1/1 -> Accumulator/1
  Delay1/1 -> Accumulator/2, Delay/1
  Convert2/1 -> Mux3/2

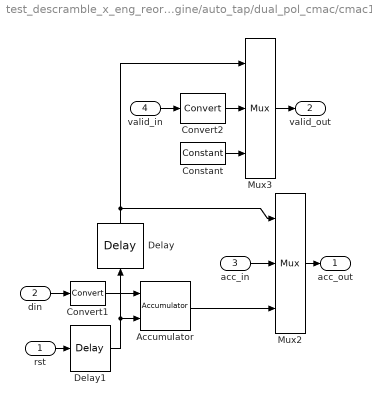
== system test_descramble_x_eng_reord/x_engine/auto_tap/dual_pol_cmac/cmac1/acc1 ==
  rst : Inport  Port=1  LatchInput=off
  din : Inport  Port=2  LatchInput=off
  acc_in : Inport  Port=3  LatchInput=off
  valid_in : Inport  Port=4  LatchInput=off
  Accumulator : xbsIndex_r3/Accumulator  n_bits=n_bits_out  overflow=Wrap  operation=Add  scale=1  explicit_period=on  period=1  rst=on  hasbypass=on  en=off  dbl_ovrd=off  show_param=off  gen_core=off  use_rpm=on
      settings: xl_area=[0, 0, 0, 0, 0, 0, 0]
  Constant : xbsIndex_r3/Constant  const=1  equ=P=C  arith_type=Boolean  n_bits=1  bin_pt=0  opselect=C  inp2=PCIN>>17  opr=+  inp1=P  carry=CIN  iostate=0  explicit_period=on  period=1  dbl_ovrd=off
  Convert1 : xbsIndex_r3/Convert  arith_type="Signed  (2's comp)"  n_bits=n_bits_out  bin_pt=2*(n_bits-1)  quantization=Truncate  overflow=Wrap  latency=0  explicit_period=off  period=1  dbl_ovrd=off  show_param=on  inserted_by_tool=off  pipeline=off
      settings: xl_area=[0, 0, 0, 0, 0, 0, 0]
  Convert2 : xbsIndex_r3/Convert  arith_type=Boolean  n_bits=8  bin_pt=6  quantization=Truncate  overflow=Wrap  latency=0  explicit_period=off  period=1  dbl_ovrd=off  show_param=off  inserted_by_tool=off  pipeline=off
      settings: xl_area=[0, 0, 0, 0, 0, 0, 0]
  Delay : xbsIndex_r3/Delay  Orientation=up  latency=0  reg_retiming=off  explicit_period=off  period=1  en=off  accept_only_valid=off  init_zero=on  dbl_ovrd=off  show_param=off
      settings: xl_area=[0, 0, 0, 0, 0, 0, 0]
  Delay1 : xbsIndex_r3/Delay  latency=0  reg_retiming=off  explicit_period=off  period=1  en=off  accept_only_valid=off  init_zero=on  dbl_ovrd=off  show_param=off
      settings: xl_area=[0, 0, 0, 0, 0, 0, 0]
  Mux2 : xbsIndex_r3/Mux  inputs=2  precision=Full  arith_type="Signed  (2's comp)"  n_bits=0  bin_pt=0  quantization="Round  (unbiased: +/- Inf)"  overflow=Wrap  latency=2  explicit_period=on  period=1  en=off  dbl_ovrd=off  show_param=off  mux_type=off  use_rpm=off  gen_core=off
      settings: xl_area=[0, 0, 0, 0, 0, 0, 0]
  Mux3 : xbsIndex_r3/Mux  inputs=2  precision=Full  arith_type="Signed  (2's comp)"  n_bits=0  bin_pt=0  quantization=Truncate  overflow=Wrap  latency=2  explicit_period=on  period=1  en=off  dbl_ovrd=off  show_param=off  mux_type=off  use_rpm=off  gen_core=off
      settings: xl_area=[0, 0, 0, 0, 0, 0, 0]
  acc_out : Outport
  valid_out : Outport  Port=2
  wires:
  Convert2/1 -> Mux3/2
  Delay1/1 -> Delay/1, Accumulator/2
  Convert1/1 -> Accumulator/1
  Delay/1 -> Mux2/1, Mux3/1
  rst/1 -> Delay1/1
  din/1 -> Convert1/1
  Mux3/1 -> valid_out/1
  Constant/1 -> Mux3/3
  valid_in/1 -> Convert2/1
  acc_in/1 -> Mux2/2
  Mux2/1 -> acc_out/1
  Accumulator/1 -> Mux2/3

== system test_descramble_x_eng_reord/x_engine/auto_tap/dual_pol_cmac/cmac1/c_to_ri ==
  In1 : Inport  Port=1  LatchInput=off
  Reinterpret : xbsIndex_r3/Reinterpret  force_arith_type=on  arith_type="Signed  (2's comp)"  force_bin_pt=on  bin_pt=n_bits - 1  force_valid=on
  Reinterpret1 : xbsIndex_r3/Reinterpret  force_arith_type=on  arith_type="Signed  (2's comp)"  force_bin_pt=on  bin_pt=n_bits - 1  force_valid=on
  Slice : xbsIndex_r3/Slice  mode=Upper Bit Location + Width  nbits=n_bits  bit1=0  base1=MSB of Input  bit0=0  base0=LSB of Input  boolean_output=off  explicit_period=off  period=1  dbl_ovrd=off
  Slice1 : xbsIndex_r3/Slice  mode=Lower Bit Location + Width  nbits=n_bits  bit1=0  base1=MSB of Input  bit0=0  base0=LSB of Input  boolean_output=off  explicit_period=off  period=1  dbl_ovrd=off
  Out1 : Outport
  Out2 : Outport  Port=2
  wires:
  In1/1 -> Slice1/1, Slice/1
  Reinterpret1/1 -> Out2/1
  Reinterpret/1 -> Out1/1
  Slice1/1 -> Reinterpret1/1
  Slice/1 -> Reinterpret/1

== system test_descramble_x_eng_reord/x_engine/auto_tap/dual_pol_cmac/cmac1/c_to_ri1 ==
  In1 : Inport  Port=1  LatchInput=off
  Reinterpret : xbsIndex_r3/Reinterpret  force_arith_type=on  arith_type="Signed  (2's comp)"  force_bin_pt=on  bin_pt=n_bits - 1  force_valid=on
  Reinterpret1 : xbsIndex_r3/Reinterpret  force_arith_type=on  arith_type="Signed  (2's comp)"  force_bin_pt=on  bin_pt=n_bits - 1  force_valid=on
  Slice : xbsIndex_r3/Slice  mode=Upper Bit Location + Width  nbits=n_bits  bit1=0  base1=MSB of Input  bit0=0  base0=LSB of Input  boolean_output=off  explicit_period=off  period=1  dbl_ovrd=off
  Slice1 : xbsIndex_r3/Slice  mode=Lower Bit Location + Width  nbits=n_bits  bit1=0  base1=MSB of Input  bit0=0  base0=LSB of Input  boolean_output=off  explicit_period=off  period=1  dbl_ovrd=off
  Out1 : Outport
  Out2 : Outport  Port=2
  wires:
  Slice/1 -> Reinterpret/1
  Slice1/1 -> Reinterpret1/1
  Reinterpret/1 -> Out1/1
  Reinterpret1/1 -> Out2/1
  In1/1 -> Slice/1, Slice1/1

== system test_descramble_x_eng_reord/x_engine/auto_tap/dual_pol_cmac/cmac1/c_to_ri2 ==
  In1 : Inport  Port=1  LatchInput=off
  Reinterpret : xbsIndex_r3/Reinterpret  force_arith_type=on  arith_type="Signed  (2's comp)"  force_bin_pt=on  bin_pt=n_bits_out - bit_growth - 3  force_valid=on
  Reinterpret1 : xbsIndex_r3/Reinterpret  force_arith_type=on  arith_type="Signed  (2's comp)"  force_bin_pt=on  bin_pt=n_bits_out - bit_growth - 3  force_valid=on
  Slice : xbsIndex_r3/Slice  mode=Upper Bit Location + Width  nbits=n_bits_out  bit1=0  base1=MSB of Input  bit0=0  base0=LSB of Input  boolean_output=off  explicit_period=off  period=1  dbl_ovrd=off
  Slice1 : xbsIndex_r3/Slice  mode=Lower Bit Location + Width  nbits=n_bits_out  bit1=0  base1=MSB of Input  bit0=0  base0=LSB of Input  boolean_output=off  explicit_period=off  period=1  dbl_ovrd=off
  Out1 : Outport
  Out2 : Outport  Port=2
  wires:
  In1/1 -> Slice1/1, Slice/1
  Reinterpret1/1 -> Out2/1
  Reinterpret/1 -> Out1/1
  Slice1/1 -> Reinterpret1/1
  Slice/1 -> Reinterpret/1

== system test_descramble_x_eng_reord/x_engine/auto_tap/dual_pol_cmac/cmac1/cmult* ==
  a : Inport  Port=1  LatchInput=off
  b : Inport  Port=2  LatchInput=off
  c : Inport  Port=3  LatchInput=off
  d : Inport  Port=4  LatchInput=off
  cmult_4bit_em* : casper_library/Multipliers/cmult_4bit_em*  mult_latency=mult_latency  add_latency=add_latency
  real : Outport
  imag : Outport  Port=2
  wires:
  a/1 -> cmult_4bit_em*/1
  b/1 -> cmult_4bit_em*/2
  c/1 -> cmult_4bit_em*/3
  d/1 -> cmult_4bit_em*/4
  cmult_4bit_em*/1 -> real/1
  cmult_4bit_em*/2 -> imag/1

== system test_descramble_x_eng_reord/x_engine/auto_tap/dual_pol_cmac/cmac1/ri_to_c ==
  In1 : Inport  Port=1  LatchInput=off
  In2 : Inport  Port=2  LatchInput=off
  Concat : xbsIndex_r3/Concat  num_inputs=2  explicit_period=off  period=1  dbl_ovrd=off
  Reinterpret : xbsIndex_r3/Reinterpret  force_arith_type=on  arith_type=Unsigned  force_bin_pt=on  bin_pt=0  force_valid=on
  Reinterpret1 : xbsIndex_r3/Reinterpret  force_arith_type=on  arith_type=Unsigned  force_bin_pt=on  bin_pt=0  force_valid=on
  Out1 : Outport
  wires:
  Reinterpret/1 -> Concat/1
  Reinterpret1/1 -> Concat/2
  In1/1 -> Reinterpret/1
  Concat/1 -> Out1/1
  In2/1 -> Reinterpret1/1

== system test_descramble_x_eng_reord/x_engine/auto_tap/dual_pol_cmac/cmac2/acc ==
  rst : Inport  Port=1  LatchInput=off
  din : Inport  Port=2  LatchInput=off
  acc_in : Inport  Port=3  LatchInput=off
  valid_in : Inport  Port=4  LatchInput=off
  Accumulator : xbsIndex_r3/Accumulator  n_bits=n_bits_out  overflow=Wrap  operation=Add  scale=1  explicit_period=on  period=1  rst=on  hasbypass=on  en=off  dbl_ovrd=off  show_param=off  gen_core=off  use_rpm=on
      settings: xl_area=[0, 0, 0, 0, 0, 0, 0]
  Constant : xbsIndex_r3/Constant  const=1  equ=P=C  arith_type=Boolean  n_bits=1  bin_pt=0  opselect=C  inp2=PCIN>>17  opr=+  inp1=P  carry=CIN  iostate=0  explicit_period=on  period=1  dbl_ovrd=off
  Convert1 : xbsIndex_r3/Convert  arith_type="Signed  (2's comp)"  n_bits=n_bits_out  bin_pt=2*(n_bits-1)  quantization=Truncate  overflow=Wrap  latency=0  explicit_period=off  period=1  dbl_ovrd=off  show_param=on  inserted_by_tool=off  pipeline=off
      settings: xl_area=[0, 0, 0, 0, 0, 0, 0]
  Convert2 : xbsIndex_r3/Convert  arith_type=Boolean  n_bits=8  bin_pt=6  quantization=Truncate  overflow=Wrap  latency=0  explicit_period=off  period=1  dbl_ovrd=off  show_param=off  inserted_by_tool=off  pipeline=off
      settings: xl_area=[0, 0, 0, 0, 0, 0, 0]
  Delay : xbsIndex_r3/Delay  Orientation=up  latency=0  reg_retiming=off  explicit_period=off  period=1  en=off  accept_only_valid=off  init_zero=on  dbl_ovrd=off  show_param=off
      settings: xl_area=[0, 0, 0, 0, 0, 0, 0]
  Delay1 : xbsIndex_r3/Delay  latency=0  reg_retiming=off  explicit_period=off  period=1  en=off  accept_only_valid=off  init_zero=on  dbl_ovrd=off  show_param=off
      settings: xl_area=[0, 0, 0, 0, 0, 0, 0]
  Mux2 : xbsIndex_r3/Mux  inputs=2  precision=Full  arith_type="Signed  (2's comp)"  n_bits=0  bin_pt=0  quantization="Round  (unbiased: +/- Inf)"  overflow=Wrap  latency=2  explicit_period=on  period=1  en=off  dbl_ovrd=off  show_param=off  mux_type=off  use_rpm=off  gen_core=off
      settings: xl_area=[0, 0, 0, 0, 0, 0, 0]
  Mux3 : xbsIndex_r3/Mux  inputs=2  precision=Full  arith_type="Signed  (2's comp)"  n_bits=0  bin_pt=0  quantization=Truncate  overflow=Wrap  latency=2  explicit_period=on  period=1  en=off  dbl_ovrd=off  show_param=off  mux_type=off  use_rpm=off  gen_core=off
      settings: xl_area=[0, 0, 0, 0, 0, 0, 0]
  acc_out : Outport
  valid_out : Outport  Port=2
  wires:
  Convert2/1 -> Mux3/2
  Delay1/1 -> Delay/1, Accumulator/2
  Convert1/1 -> Accumulator/1
  Delay/1 -> Mux2/1, Mux3/1
  rst/1 -> Delay1/1
  din/1 -> Convert1/1
  Mux3/1 -> valid_out/1
  Constant/1 -> Mux3/3
  valid_in/1 -> Convert2/1
  acc_in/1 -> Mux2/2
  Mux2/1 -> acc_out/1
  Accumulator/1 -> Mux2/3

== system test_descramble_x_eng_reord/x_engine/auto_tap/dual_pol_cmac/cmac2/acc1 ==
  rst : Inport  Port=1  LatchInput=off
  din : Inport  Port=2  LatchInput=off
  acc_in : Inport  Port=3  LatchInput=off
  valid_in : Inport  Port=4  LatchInput=off
  Accumulator : xbsIndex_r3/Accumulator  n_bits=n_bits_out  overflow=Wrap  operation=Add  scale=1  explicit_period=on  period=1  rst=on  hasbypass=on  en=off  dbl_ovrd=off  show_param=off  gen_core=off  use_rpm=on
      settings: xl_area=[0, 0, 0, 0, 0, 0, 0]
  Constant : xbsIndex_r3/Constant  const=1  equ=P=C  arith_type=Boolean  n_bits=1  bin_pt=0  opselect=C  inp2=PCIN>>17  opr=+  inp1=P  carry=CIN  iostate=0  explicit_period=on  period=1  dbl_ovrd=off
  Convert1 : xbsIndex_r3/Convert  arith_type="Signed  (2's comp)"  n_bits=n_bits_out  bin_pt=2*(n_bits-1)  quantization=Truncate  overflow=Wrap  latency=0  explicit_period=off  period=1  dbl_ovrd=off  show_param=on  inserted_by_tool=off  pipeline=off
      settings: xl_area=[0, 0, 0, 0, 0, 0, 0]
  Convert2 : xbsIndex_r3/Convert  arith_type=Boolean  n_bits=8  bin_pt=6  quantization=Truncate  overflow=Wrap  latency=0  explicit_period=off  period=1  dbl_ovrd=off  show_param=off  inserted_by_tool=off  pipeline=off
      settings: xl_area=[0, 0, 0, 0, 0, 0, 0]
  Delay : xbsIndex_r3/Delay  Orientation=up  latency=0  reg_retiming=off  explicit_period=off  period=1  en=off  accept_only_valid=off  init_zero=on  dbl_ovrd=off  show_param=off
      settings: xl_area=[0, 0, 0, 0, 0, 0, 0]
  Delay1 : xbsIndex_r3/Delay  latency=0  reg_retiming=off  explicit_period=off  period=1  en=off  accept_only_valid=off  init_zero=on  dbl_ovrd=off  show_param=off
      settings: xl_area=[0, 0, 0, 0, 0, 0, 0]
  Mux2 : xbsIndex_r3/Mux  inputs=2  precision=Full  arith_type="Signed  (2's comp)"  n_bits=0  bin_pt=0  quantization="Round  (unbiased: +/- Inf)"  overflow=Wrap  latency=2  explicit_period=on  period=1  en=off  dbl_ovrd=off  show_param=off  mux_type=off  use_rpm=off  gen_core=off
      settings: xl_area=[0, 0, 0, 0, 0, 0, 0]
  Mux3 : xbsIndex_r3/Mux  inputs=2  precision=Full  arith_type="Signed  (2's comp)"  n_bits=0  bin_pt=0  quantization=Truncate  overflow=Wrap  latency=2  explicit_period=on  period=1  en=off  dbl_ovrd=off  show_param=off  mux_type=off  use_rpm=off  gen_core=off
      settings: xl_area=[0, 0, 0, 0, 0, 0, 0]
  acc_out : Outport
  valid_out : Outport  Port=2
  wires:
  Accumulator/1 -> Mux2/3
  Mux2/1 -> acc_out/1
  acc_in/1 -> Mux2/2
  valid_in/1 -> Convert2/1
  Constant/1 -> Mux3/3
  Mux3/1 -> valid_out/1
  din/1 -> Convert1/1
  rst/1 -> Delay1/1
  Delay/1 -> Mux3/1, Mux2/1
  Convert1/1 -> Accumulator/1
  Delay1/1 -> Accumulator/2, Delay/1
  Convert2/1 -> Mux3/2

== system test_descramble_x_eng_reord/x_engine/auto_tap/dual_pol_cmac/cmac2/c_to_ri ==
  In1 : Inport  Port=1  LatchInput=off
  Reinterpret : xbsIndex_r3/Reinterpret  force_arith_type=on  arith_type="Signed  (2's comp)"  force_bin_pt=on  bin_pt=n_bits - 1  force_valid=on
  Reinterpret1 : xbsIndex_r3/Reinterpret  force_arith_type=on  arith_type="Signed  (2's comp)"  force_bin_pt=on  bin_pt=n_bits - 1  force_valid=on
  Slice : xbsIndex_r3/Slice  mode=Upper Bit Location + Width  nbits=n_bits  bit1=0  base1=MSB of Input  bit0=0  base0=LSB of Input  boolean_output=off  explicit_period=off  period=1  dbl_ovrd=off
  Slice1 : xbsIndex_r3/Slice  mode=Lower Bit Location + Width  nbits=n_bits  bit1=0  base1=MSB of Input  bit0=0  base0=LSB of Input  boolean_output=off  explicit_period=off  period=1  dbl_ovrd=off
  Out1 : Outport
  Out2 : Outport  Port=2
  wires:
  Slice/1 -> Reinterpret/1
  Slice1/1 -> Reinterpret1/1
  Reinterpret/1 -> Out1/1
  Reinterpret1/1 -> Out2/1
  In1/1 -> Slice/1, Slice1/1

== system test_descramble_x_eng_reord/x_engine/auto_tap/dual_pol_cmac/cmac2/c_to_ri1 ==
  In1 : Inport  Port=1  LatchInput=off
  Reinterpret : xbsIndex_r3/Reinterpret  force_arith_type=on  arith_type="Signed  (2's comp)"  force_bin_pt=on  bin_pt=n_bits - 1  force_valid=on
  Reinterpret1 : xbsIndex_r3/Reinterpret  force_arith_type=on  arith_type="Signed  (2's comp)"  force_bin_pt=on  bin_pt=n_bits - 1  force_valid=on
  Slice : xbsIndex_r3/Slice  mode=Upper Bit Location + Width  nbits=n_bits  bit1=0  base1=MSB of Input  bit0=0  base0=LSB of Input  boolean_output=off  explicit_period=off  period=1  dbl_ovrd=off
  Slice1 : xbsIndex_r3/Slice  mode=Lower Bit Location + Width  nbits=n_bits  bit1=0  base1=MSB of Input  bit0=0  base0=LSB of Input  boolean_output=off  explicit_period=off  period=1  dbl_ovrd=off
  Out1 : Outport
  Out2 : Outport  Port=2
  wires:
  In1/1 -> Slice1/1, Slice/1
  Reinterpret1/1 -> Out2/1
  Reinterpret/1 -> Out1/1
  Slice1/1 -> Reinterpret1/1
  Slice/1 -> Reinterpret/1

== system test_descramble_x_eng_reord/x_engine/auto_tap/dual_pol_cmac/cmac2/c_to_ri2 ==
  In1 : Inport  Port=1  LatchInput=off
  Reinterpret : xbsIndex_r3/Reinterpret  force_arith_type=on  arith_type="Signed  (2's comp)"  force_bin_pt=on  bin_pt=n_bits_out - bit_growth - 3  force_valid=on
  Reinterpret1 : xbsIndex_r3/Reinterpret  force_arith_type=on  arith_type="Signed  (2's comp)"  force_bin_pt=on  bin_pt=n_bits_out - bit_growth - 3  force_valid=on
  Slice : xbsIndex_r3/Slice  mode=Upper Bit Location + Width  nbits=n_bits_out  bit1=0  base1=MSB of Input  bit0=0  base0=LSB of Input  boolean_output=off  explicit_period=off  period=1  dbl_ovrd=off
  Slice1 : xbsIndex_r3/Slice  mode=Lower Bit Location + Width  nbits=n_bits_out  bit1=0  base1=MSB of Input  bit0=0  base0=LSB of Input  boolean_output=off  explicit_period=off  period=1  dbl_ovrd=off
  Out1 : Outport
  Out2 : Outport  Port=2
  wires:
  Slice/1 -> Reinterpret/1
  Slice1/1 -> Reinterpret1/1
  Reinterpret/1 -> Out1/1
  Reinterpret1/1 -> Out2/1
  In1/1 -> Slice/1, Slice1/1

== system test_descramble_x_eng_reord/x_engine/auto_tap/dual_pol_cmac/cmac2/cmult* ==
  a : Inport  Port=1  LatchInput=off
  b : Inport  Port=2  LatchInput=off
  c : Inport  Port=3  LatchInput=off
  d : Inport  Port=4  LatchInput=off
  cmult_4bit_em* : casper_library/Multipliers/cmult_4bit_em*  mult_latency=mult_latency  add_latency=add_latency
  real : Outport
  imag : Outport  Port=2
  wires:
  a/1 -> cmult_4bit_em*/1
  b/1 -> cmult_4bit_em*/2
  c/1 -> cmult_4bit_em*/3
  d/1 -> cmult_4bit_em*/4
  cmult_4bit_em*/1 -> real/1
  cmult_4bit_em*/2 -> imag/1
